simulink model "fixpt_sl_product_mul_hdl"  (Simulink 7.9)
settings: Solver=FixedStepDiscrete  SolverMode=SingleTasking  StartTime=0.0  StopTime=10.0  RelTol=1e-3
settings Model: Creator=at-mt  LastModifiedBy=amatsumo
settings DataIOCC: SaveOutput=off  SignalLogging=off  SaveTime=off
settings OptimizationCC: BlockReduction=off  ConditionallyExecuteInputs=off  InlineParams=on  InitFltsAndDblsToZero=on
settings DebuggingCC: AlgebraicLoopMsg=error  SingleTaskRateTransMsg=error  FcnCallInpInsideContextMsg=Use local settings  StrictBusMsg=Warning
settings HardwareCC: ProdHWDeviceType=ASIC/FPGA->ASIC/FPGA  TargetEndianess=LittleEndian  TargetHWDeviceType=MATLAB Host  ProdEqTarget=off
settings GRTTargetCC: CombineOutputUpdateFcns=off  GRTInterface=on

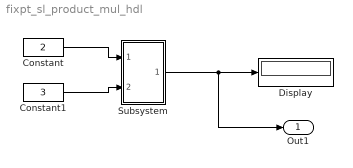
== system fixpt_sl_product_mul_hdl ==
  Constant : Constant  Value=2  OutDataTypeStr=fixdt(1,8,1)  SampleTime=1
      settings: AttributesFormatString=DataType = %<OutDataTypeStr>
  Constant1 : Constant  Value=3  OutDataTypeStr=fixdt(1,8,2)  SampleTime=1
      settings: AttributesFormatString=DataType = %<OutDataTypeStr>
  Display : Display
      settings: AttributesFormatString=Format = %<Format>
  Subsystem : Subsystem
  Out1 : Outport
  wires:
  Subsystem/1(Out1) -> Out1/1, Display/1
  Constant/1 -> Subsystem/1(In1)
  Constant1/1 -> Subsystem/2(In2)

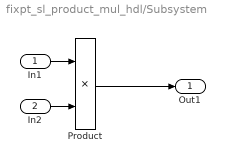
== system fixpt_sl_product_mul_hdl/Subsystem ==
  In1 : Inport
  In2 : Inport  Port=2
  Product : Product  OutDataTypeStr=fixdt(1,14,1)  RndMeth=Zero
  Out1 : Outport
  wires:
  In2/1 -> Product/2
  Product/1 -> Out1/1
  In1/1 -> Product/1
